simulink model "direct_form2_withsub"  (R2014b)
settings: Solver=ode45  StartTime=0.0  StopTime=10.0  RelTol=1e-3
settings Model: Creator=ravoson  LastModifiedBy=ravoson

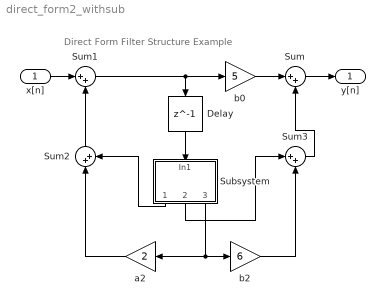
== system direct_form2_withsub ==
  note: Direct Form Filter Structure Example
  x[n] : Inport
  Delay : Delay  DelayLength=1  InitialCondition=0
  Subsystem : Subsystem
  Sum{,1..3} (4 alike) : Sum  Inputs=|++
  a2 : Gain  Gain=2
  b0 : Gain  Gain=5
  b2 : Gain  Gain=6
  y[n] : Outport
  wires:
  x[n]/1 -> Sum1/1
  Sum1/1 -> Delay/1, b0/1
  b0/1 -> Sum/1
  Sum/1 -> y[n]/1
  Sum2/1 -> Sum1/2
  a2/1 -> Sum2/1
  Sum3/1 -> Sum/2
  b2/1 -> Sum3/2
  Subsystem/3(Out3) -> b2/1, a2/1
  Delay/1 -> Subsystem/1(In1)
  Subsystem/1(Out1) -> Sum2/2
  Subsystem/2(Out2) -> Sum3/1

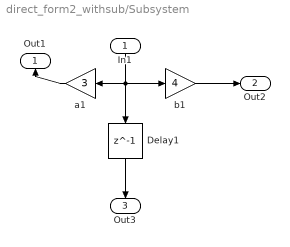
== system direct_form2_withsub/Subsystem ==
  In1 : Inport
  Delay1 : Delay  DelayLength=1  InitialCondition=0
  a1 : Gain  Gain=3
  b1 : Gain  Gain=4
  Out1 : Outport
  Out2 : Outport  Port=2
  Out3 : Outport  Port=3
  wires:
  b1/1 -> Out2/1
  a1/1 -> Out1/1
  Delay1/1 -> Out3/1
  In1/1 -> Delay1/1, b1/1, a1/1
